simulink model "Reshape_TestGen8"  (R2017b)
settings: Solver=FixedStepDiscrete  StartTime=0.0  StopTime=10.0  RelTol=1e-3
undefined symbols (not defined in the file): Block_TestLib, reset
settings Model: Creator=ktrinh  LastModifiedBy=ktrinh
settings DebuggingCC: ParameterOverflowMsg=none

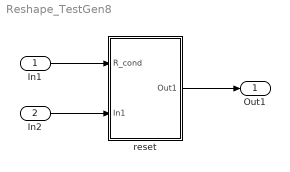
== system Reshape_TestGen8 ==
  In1 : Inport
  In2 : Inport  Port=2
  reset : Subsystem  AncestorBlock=Block_TestLib/reset
  Out1 : Outport
  wires:
  In1/1 -> reset/1(R_cond)
  In2/1 -> reset/2(In1)
  reset/1(Out1) -> Out1/1

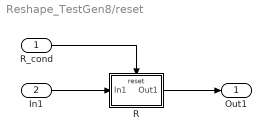
== system Reshape_TestGen8/reset ==
  R_cond : Inport  OutDataTypeStr=boolean
  In1 : Inport  Port=2
  R : Subsystem  TreatAsAtomicUnit=on
  Out1 : Outport
  wires:
  R_cond/1 -> R/Reset
  In1/1 -> R/1(In1)
  R/1(Out1) -> Out1/1

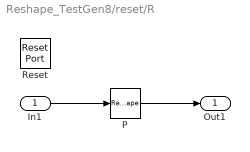
== system Reshape_TestGen8/reset/R ==
  In1 : Inport  OutDataTypeStr=int8  PortDimensions=[2,3]
  Reset : ResetPort  DisableCoverage=on
  P : Reshape  OutputDimensionality=Column vector (2-D)
  Out1 : Outport
  wires:
  In1/1 -> P/1
  P/1 -> Out1/1
